simulink model "ParallelAssemblyEstimation2"  (R2024a)
settings: Solver=VariableStepAuto  StartTime=0.0  StopTime=10*10000  FixedStep=Ts  RelTol=1e-3  EnableMultiTasking=on
PreLoadFcn:
  | BatterySOHEstimationData;
values from neighbouring files (symbols this model uses):
  BalThreshold = 0.005    [ParallelAssemblyEstimationData.m]
  Ki = 10    [ParallelAssemblyEstimationData.m]
  Kp = 100    [ParallelAssemblyEstimationData.m]
  R = 0.05    [ParallelAssemblyEstimationData.m]
  R00 = 0.008    [ParallelAssemblyEstimationData.m]
  R0_mat = [.0117, .0085, .009; .011, .0085, .009; .0114, .0087, .0092; .0107, .0082, .0088; .0107, .0083, .0091; .0113, .0085, .0089; .0116, .0085, .0089]    [ParallelAssemblyEstimationData.m]
  SOC0 = initialSOC    (= 0.1)    [ParallelAssemblyEstimationData.m]
  Ts = 1    [ParallelAssemblyEstimationData.m]
libraries: nesl_utility x9, fl_lib x8, simulink x2, BatteryEstimators x2, BatteryCurrentManagement x1, BatteryBalancing x1, PouchCellAMP20M1HD x1, PouchCellAMP20M1HD_2 x1
CloseFcn:
  | try
  |     close(h1_BatterySOHEstimation)
  | catch
  | end
  | 
  | clear h1_BatterySOHEstimation
  | 
  | clear BatterySOHEstimationSimlog
  | clear BatterySOHEstimationLogsout
  | 
  | clear AH SOC_vec T_vec R0_mat R1_mat tau1_mat
  | clear V0_mat Q R P0 initialSOC SOC0 R00 Ts
  | clear cell_area h_conv thermal_mass
Description:
  | Battery State-of-Health Estimation
settings Model: Creator=The MathWorks, Inc.  LastModifiedBy=Carlos
settings SolverCC: AlgebraicLoopSolver=TrustRegion  AutoInsertRateTranBlk=on  MaxZcPerStep=1
settings DataIOCC: MaxDataPoints=370000  ReturnWorkspaceOutputs=off  SignalLoggingName=BatterySOHEstimationLogsout
settings OptimizationCC: ReuseModelBlockBuffer=off  LifeSpan=inf
settings DebuggingCC: UnconnectedInputMsg=warning  UnconnectedOutputMsg=warning  UnconnectedLineMsg=warning  SFUnexpectedBacktrackingDiag=warning  SFNoUnconditionalDefaultTransitionDiag=warning  SFExecutionAtInitializationDiag=none  ArithmeticOperatorsInVariantConditions=warning
settings ModelReferenceCC: EnableRefExpFcnMdlSchedulingChecks=on
settings SFSimCC: SimUseLocalCustomCode=off  CustomCodeUndefinedFunction=UseInterfaceOnly
settings RTWCC: RTWUseLocalCustomCode=off  GPUComputeCapability=3.5  DLArmComputeVersion=19.05
settings CodeAppCC: StateflowObjectComments=on
settings GRTTargetCC: TargetLangStandard=C89/C90 (ANSI)
settings ConfigComp: CovMetricSettings=dw  CovSaveCumulativeToWorkspaceVar=on  CovSaveSingleToWorkspaceVar=on  CovExternalEMLEnable=off
settings SimscapeCC: SimscapeLogType=all  SimscapeLogSimulationStatistics=on  SimscapeLogName=BatterySOHEstimationSimlog  SimscapeLogDataHistory=370000

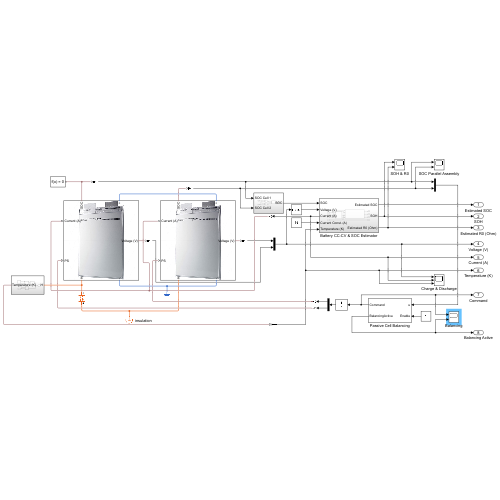
[thumbnail: Simulink's stored preview of the top-level diagram]
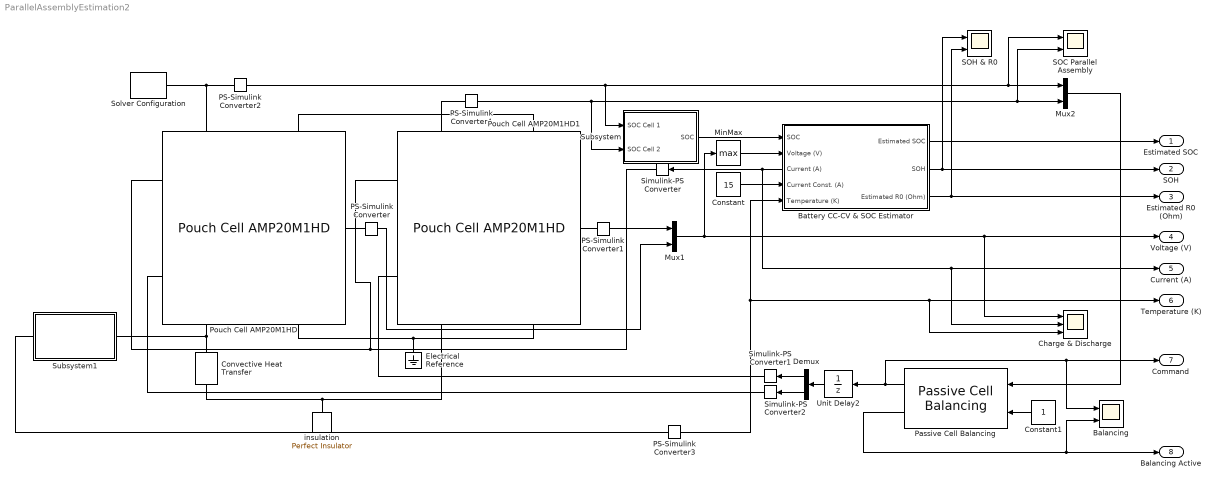
== system ParallelAssemblyEstimation2 ==
  Balancing : Scope  NumInputPorts=2
  Battery CC-CV & SOC Estimator : Subsystem
      settings: PortSchema="{\"entries\":[{\"content\":{\"sides\":[{\"content\":{\"connectorIds\":[\"In1\",\"In2\",\"Out4\",\"In3\",\"In4\"]},\"type\":\"ConnectorPlacement.EquallySpacedRectSide\",\"uuid\":\"2514b7b4-00c3-492f-9a2e-50aa1b82d6f8\"},{\"content\":{\"connectorIds\":[\"Out1\",\"Out2\",\"Out3\"],\"side\":\"RIGHT\"},\"type\":\"ConnectorPlacement.EquallySpacedRectSide\",\"uuid\":\"cd4e48b2-778c-43ee-9be2-ddbae3415521\"},{\"content\":{\"side\":\"TOP\"},\"type\":\"ConnectorPlacement.EquallySpacedRectSide\",\"uuid\":\"5acb0ed7-42f7-4cae-ae5e-6504fab96612\"}]},\"type\":\"ConnectorPlacement.EquallySpacedConnector\",\"uuid\":\"df921565-b99f-40a9-8d77-9b2ba5142a69\"}],\"packageUris\":[\"http://schema.mathworks.com/mf0/Connector/R2020b\"],\"version\":\"1.0\"}"
  Charge & Discharge : Scope  NumInputPorts=3
  Constant : Constant  Value=15
  Constant1 : Constant
  Convective Heat Transfer : fl_lib/Thermal/Thermal Elements/Convective Heat Transfer  thermal_type=foundation.enum.constant_variable.constant  area=cell_area m^2  heat_tr_coeff=h_conv W/(K*m^2)  min_heat_tr_coeff=1e-3 W/(K*m^2)  T_specify=off  T_priority=None  T=0 K  T_nominal_specify=off  T_nominal_value=1  T_nominal_unit=K  Q_specify=off  Q_priority=None  Q=0 W  Q_nominal_specify=off  Q_nominal_value=1  Q_nominal_unit=W
  Demux : Demux  Outputs=2
  Electrical Reference : fl_lib/Electrical/Electrical Elements/Electrical Reference
  MinMax : MinMax  Function=max
  Mux1 : Mux  Inputs=2
  Mux2 : Mux  Inputs=2
  PS-Simulink Converter{,1..4} (5 alike) : nesl_utility/PS-Simulink Converter  PhysicalDomain=network_engine_domain  SubClassName=ps_output  LeftPortType=input  RightPortType=output  PseudoPeriodic=off  Frequencies=[]  VectorFormat=inherit  Unit=inherit  AffineConversion=off
  Passive Cell Balancing : BatteryBalancing/Passive Cell Balancing  Threshold=BalThreshold  HysteresisBand=0  Td_on=1  Td_off=1  Ts=Ts  dataType=double
      settings: LibrarySourceBlock=batt_sl_lib/Cell Balancing/Passive Cell Balancing
  Pouch Cell AMP20M1HD : PouchCellAMP20M1HD/Pouch Cell AMP20M1HD  SystemSampleTime=-1  VariantActivationTime=update diagram  AllowFlexibleInterface=on  Latency=0  AutoFrameSizeCalculation=off
      settings: PortSchema="{\"entries\":[{\"content\":{\"sides\":[{\"content\":{\"connectorIds\":[\"LConn1\",\"LConn2\"]},\"type\":\"ConnectorPlacement.EquallySpacedRectSide\",\"uuid\":\"1ad4bd77-f3cd-4a33-b1f1-8549cde45efa\"},{\"content\":{\"connectorIds\":[\"RConn1\"],\"side\":\"RIGHT\"},\"type\":\"ConnectorPlacement.EquallySpacedRectSide\",\"uuid\":\"9571ac2f-f2ec-4c0a-999c-8ea72e2cf4ad\"},{\"content\":{\"connectorIds\":[\"LConn3\",\"LConn4\"],\"side\":\"TOP\"},\"type\":\"ConnectorPlacement.EquallySpacedRectSide\",\"uuid\":\"d345a9ac-e4a8-4cf5-b4f6-097232c3cb5c\"},{\"content\":{\"connectorIds\":[\"RConn2\",\"RConn3\"],\"side\":\"BOTTOM\"},\"type\":\"ConnectorPlacement.EquallySpacedRectSide\",\"uuid\":\"7baf50c1-841c-4e4e-b39d-add364b405c0\"}]},\"type\":\"ConnectorPlacement.EquallySpacedConnector\",\"uuid\":\"1a2d2ccb-b2c1-437b-8298-ee46cad3b357\"}],\"packageUris\":[\"http://schema.mathworks.com/mf0/Connector/R2020b\"],\"version\":\"1.0\"}"
  Pouch Cell AMP20M1HD1 : PouchCellAMP20M1HD_2/Pouch Cell AMP20M1HD  SystemSampleTime=-1  VariantActivationTime=update diagram  AllowFlexibleInterface=on  Latency=0  AutoFrameSizeCalculation=off
      settings: PortSchema="{\"entries\":[{\"content\":{\"sides\":[{\"content\":{\"connectorIds\":[\"LConn1\",\"LConn2\"]},\"type\":\"ConnectorPlacement.EquallySpacedRectSide\",\"uuid\":\"1ad4bd77-f3cd-4a33-b1f1-8549cde45efa\"},{\"content\":{\"connectorIds\":[\"RConn1\"],\"side\":\"RIGHT\"},\"type\":\"ConnectorPlacement.EquallySpacedRectSide\",\"uuid\":\"9571ac2f-f2ec-4c0a-999c-8ea72e2cf4ad\"},{\"content\":{\"connectorIds\":[\"LConn3\",\"LConn4\"],\"side\":\"TOP\"},\"type\":\"ConnectorPlacement.EquallySpacedRectSide\",\"uuid\":\"d345a9ac-e4a8-4cf5-b4f6-097232c3cb5c\"},{\"content\":{\"connectorIds\":[\"RConn2\",\"RConn3\"],\"side\":\"BOTTOM\"},\"type\":\"ConnectorPlacement.EquallySpacedRectSide\",\"uuid\":\"7baf50c1-841c-4e4e-b39d-add364b405c0\"}]},\"type\":\"ConnectorPlacement.EquallySpacedConnector\",\"uuid\":\"1a2d2ccb-b2c1-437b-8298-ee46cad3b357\"}],\"packageUris\":[\"http://schema.mathworks.com/mf0/Connector/R2020b\"],\"version\":\"1.0\"}"
  SOC Parallel Assembly : Scope  NumInputPorts=2
  SOH & R0 : Scope  NumInputPorts=2
  Simulink-PS Converter : nesl_utility/Simulink-PS Converter  PhysicalDomain=network_engine_domain  SubClassName=ps_input  LeftPortType=input  RightPortType=output  PseudoPeriodic=off  Frequencies=[]  NoiseDistribution=none  NoiseParameters=[]  Unit=1  AffineConversion=off  FilteringAndDerivatives=provide  SimscapeFilterOrder=1  InputFilterTimeConstant=0.001  UdotUserProvided=0
  Simulink-PS Converter1 : nesl_utility/Simulink-PS Converter  PhysicalDomain=network_engine_domain  SubClassName=ps_input  LeftPortType=input  RightPortType=output  PseudoPeriodic=off  Frequencies=[]  NoiseDistribution=none  NoiseParameters=[]  Unit=1  AffineConversion=off  FilteringAndDerivatives=provide  SimscapeFilterOrder=1  InputFilterTimeConstant=0.001  UdotUserProvided=0
  Simulink-PS Converter2 : nesl_utility/Simulink-PS Converter  PhysicalDomain=network_engine_domain  SubClassName=ps_input  LeftPortType=input  RightPortType=output  PseudoPeriodic=off  Frequencies=[]  NoiseDistribution=none  NoiseParameters=[]  Unit=1  AffineConversion=off  FilteringAndDerivatives=provide  SimscapeFilterOrder=1  InputFilterTimeConstant=0.001  UdotUserProvided=0
  Solver Configuration : nesl_utility/Solver Configuration  PhysicalDomain=network_engine_domain  SubClassName=solver  LeftPortType=input  RightPortType=generic  Tones=[]  Harmonics=[]  SimulateNoise=off  Profile=off  UseLocalSampling=off  EnableSwitchedLinearOptims=on  FrequencyDomain=off  UseCCode=off  RelTol=0.001  AbsTol=0.001  MinStep=1e-09  ToWorkspace=off  RevertToSquareIcSolve=off  NumHomotopyIterations=100  PhasorMode=off  PhasorModeNumHarmonics=1  ConsistencySolver=NEWTON_XTOL_AFTER_FTOL  IndexReductionMethod=DerivativeReplacement  DoDC=off  ResidualTolerance=1e-09  ConsistencyTolSource=GLOBAL  ConsistencyAbsTol=0.001  ConsistencyRelTol=0.001  ConsistencyTolFactor=0.001  UseLocalSolver=on  LocalSolverChoice=NE_BACKWARD_EULER_ADVANCER  ResolveIndetEquations=on  FunctionEvalNumThread=1  LocalSolverSampleTime=Ts  DoFixedCost=on  MaxNonlinIter=3  MaxModeIter=2  ComputeImpulses=off  ImpulseIterations=2  LinearAlgebra=auto  LinearAlgebraNumThread=0  EquationFormulation=NE_TIME_EF  DelaysMemoryBudget=1024  AutomaticFiltering=on  FilteringTimeConstant=0.001  PartitionStorageMethod=AS_NEEDED  PartitionMemoryBudget=1024  PartitionMethod=ROBUST  MultibodyUseLocalSolver=off  MultibodyLocalSolverChoice=ODE1  MultibodyLocalSolverSampleTime=0.001
  Subsystem : Subsystem
  Subsystem1 : Subsystem
  Unit Delay2 : UnitDelay  SampleTime=-1  HasFrameUpgradeWarning=on
  insulation : fl_lib/Thermal/Thermal Elements/Perfect Insulator  T_specify=off  T_priority=None  T=0 K  T_nominal_specify=off  T_nominal_value=1  T_nominal_unit=K
  Estimated SOC : Outport
  SOH : Outport  Port=2
  Estimated R0 (Ohm) : Outport  Port=3
  Voltage (V) : Outport  Port=4
  Current (A) : Outport  Port=5
  Temperature (K) : Outport  Port=6
  Command : Outport  Port=7
  Balancing Active : Outport  Port=8
  wires:
  Battery CC-CV & SOC Estimator/2(SOH) -> SOH/1, SOH & R0/1
  Battery CC-CV & SOC Estimator/3(Estimated R0 (Ohm)) -> Estimated R0 (Ohm)/1, SOH & R0/2
  Battery CC-CV & SOC Estimator/1(Estimated SOC) -> Estimated SOC/1
  Constant/1 -> Battery CC-CV & SOC Estimator/3(Current Const. (A))
  Battery CC-CV & SOC Estimator/4(Current (A)) -> Simulink-PS Converter/1, Charge & Discharge/2, Current (A)/1
  PS-Simulink Converter/1 -> Mux1/2
  Mux1/1 -> MinMax/1, Voltage (V)/1, Charge & Discharge/1
  PS-Simulink Converter4/1 -> Mux2/2, SOC Parallel Assembly/2, Subsystem/2(SOC Cell 2)
  PS-Simulink Converter2/1 -> SOC Parallel Assembly/1, Mux2/1, Subsystem/1(SOC Cell 1)
  Unit Delay2/1 -> Demux/1
  Passive Cell Balancing/1 -> Unit Delay2/1, Command/1, Balancing/1
  Passive Cell Balancing/2 -> Balancing Active/1, Balancing/2
  Demux/1 -> Simulink-PS Converter1/1
  Demux/2 -> Simulink-PS Converter2/1
  Constant1/1 -> Passive Cell Balancing/2
  MinMax/1 -> Battery CC-CV & SOC Estimator/2(Voltage (V))
  PS-Simulink Converter3/1 -> Temperature (K)/1, Charge & Discharge/3, Battery CC-CV & SOC Estimator/4(Temperature (K))
  PS-Simulink Converter1/1 -> Mux1/1
  Mux2/1 -> Passive Cell Balancing/1
  Subsystem/1(SOC) -> Battery CC-CV & SOC Estimator/1(SOC)
  connections:
  Pouch Cell AMP20M1HD/LConn4 -- Pouch Cell AMP20M1HD1/LConn4
  Electrical Reference/LConn1 -- Pouch Cell AMP20M1HD1/RConn3 -- Pouch Cell AMP20M1HD/RConn3
  Pouch Cell AMP20M1HD/RConn1 -- PS-Simulink Converter/LConn1
  PS-Simulink Converter1/LConn1 -- Pouch Cell AMP20M1HD1/RConn1
  PS-Simulink Converter2/LConn1 -- Solver Configuration/RConn1 -- Pouch Cell AMP20M1HD/LConn3
  PS-Simulink Converter4/LConn1 -- Pouch Cell AMP20M1HD1/LConn3
  Simulink-PS Converter/RConn1 -- Pouch Cell AMP20M1HD1/LConn1 -- Pouch Cell AMP20M1HD/LConn1
  Pouch Cell AMP20M1HD/RConn2 -- Convective Heat Transfer/LConn1 -- Subsystem1/RConn1
  Pouch Cell AMP20M1HD1/LConn2 -- Simulink-PS Converter1/RConn1
  Pouch Cell AMP20M1HD/LConn2 -- Simulink-PS Converter2/RConn1
  PS-Simulink Converter3/LConn1 -- Subsystem1/LConn1
  insulation/LConn1 -- Pouch Cell AMP20M1HD1/RConn2 -- Convective Heat Transfer/RConn1

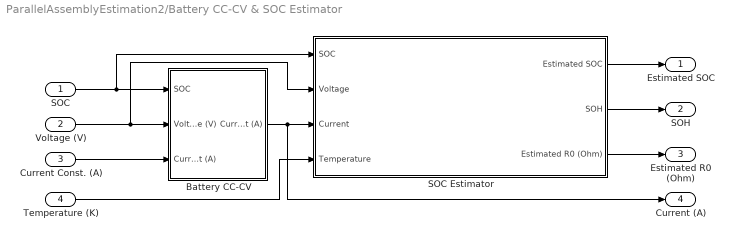
== system ParallelAssemblyEstimation2/Battery CC-CV & SOC Estimator ==
  SOC : Inport
  Voltage (V) : Inport  Port=2
  Current Const. (A) : Inport  Port=3
  Temperature (K) : Inport  Port=4
  Battery CC-CV : Subsystem
  SOC Estimator : Subsystem
  Estimated SOC : Outport
  SOH : Outport  Port=2
  Estimated R0 (Ohm) : Outport  Port=3
  Current (A) : Outport  Port=4
  wires:
  Temperature (K)/1 -> SOC Estimator/4(Temperature)
  Battery CC-CV/1(Current Out (A)) -> SOC Estimator/3(Current), Current (A)/1
  SOC Estimator/2(SOH) -> SOH/1
  SOC Estimator/3(Estimated R0 (Ohm)) -> Estimated R0 (Ohm)/1
  SOC Estimator/1(Estimated SOC) -> Estimated SOC/1
  Current Const. (A)/1 -> Battery CC-CV/3(Current (A))
  Voltage (V)/1 -> SOC Estimator/2(Voltage), Battery CC-CV/2(Voltage (V))
  SOC/1 -> SOC Estimator/1(SOC), Battery CC-CV/1(SOC)

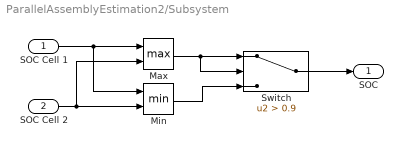
== system ParallelAssemblyEstimation2/Subsystem ==
  SOC Cell 1 : Inport
  SOC Cell 2 : Inport  Port=2
  Max : MinMax  Function=max  Inputs=2
  Min : MinMax  Inputs=2
  Switch : Switch  Criteria=u2 > Threshold  Threshold=0.9  SaturateOnIntegerOverflow=off  InputSameDT=off
  SOC : Outport
  wires:
  SOC Cell 1/1 -> Max/1, Min/1
  Max/1 -> Switch/1, Switch/2
  Min/1 -> Switch/3
  SOC Cell 2/1 -> Max/2, Min/2
  Switch/1 -> SOC/1

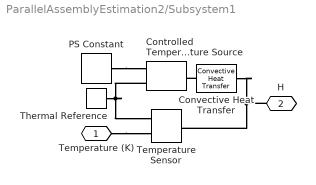
== system ParallelAssemblyEstimation2/Subsystem1 ==
  Controlled Temperature Source : fl_lib/Thermal/Thermal Sources/Controlled Temperature Source
  Convective Heat Transfer : fl_lib/Thermal/Thermal Elements/Convective Heat Transfer  thermal_type=foundation.enum.constant_variable.constant  area=cell_area m^2  heat_tr_coeff=h_conv W/(K*m^2)  min_heat_tr_coeff=1e-3 W/(K*m^2)  T_specify=off  T_priority=None  T=0 K  T_nominal_specify=off  T_nominal_value=1  T_nominal_unit=K  Q_specify=off  Q_priority=None  Q=0 W  Q_nominal_specify=off  Q_nominal_value=1  Q_nominal_unit=W
  PS Constant : fl_lib/Physical Signals/Sources/PS Constant  constant=cell_temperature K
  Temperature Sensor : fl_lib/Thermal/Thermal Sensors/Temperature Sensor  temperature_measure=foundation.enum.MeasurementReference.difference
  Thermal Reference : fl_lib/Thermal/Thermal Elements/Thermal Reference
  Temperature (K) : PMIOPort  Side=Left
  H : PMIOPort  Port=2  Side=Right
  connections:
  H/RConn1 -- Convective Heat Transfer/RConn1 -- Temperature Sensor/LConn1
  Thermal Reference/LConn1 -- Controlled Temperature Source/RConn2 -- Temperature Sensor/RConn1
  PS Constant/RConn1 -- Controlled Temperature Source/RConn1
  Temperature (K)/RConn1 -- Temperature Sensor/RConn2
  Convective Heat Transfer/LConn1 -- Controlled Temperature Source/LConn1

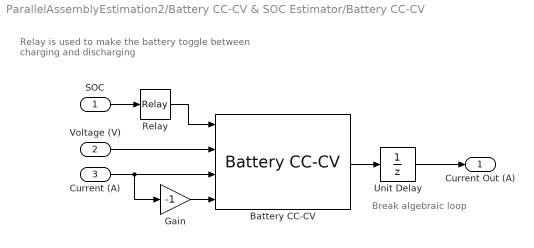
== system ParallelAssemblyEstimation2/Battery CC-CV & SOC Estimator/Battery CC-CV ==
  note: Break algebraic loop
  note: Relay is used to make the battery toggle between charging and discharging
  SOC : Inport
  Voltage (V) : Inport  Port=2
  Current (A) : Inport  Port=3
  Battery CC-CV : BatteryCurrentManagement/Battery CC-CV  MaxCellVoltage=vMax  Kp=Kp  Ki=Ki  Kaw=Kaw  Kt=1  Ts=Ts
      settings: LibrarySourceBlock=batt_sl_lib/Current Management/Battery CC-CV
  Gain : Gain  Gain=-1
  Relay : Relay  OnSwitchValue=0.9186  OffSwitchValue=0.3  OnOutputValue=0  OffOutputValue=1
  Unit Delay : UnitDelay  SampleTime=-1  HasFrameUpgradeWarning=on
  Current Out (A) : Outport
  wires:
  Voltage (V)/1 -> Battery CC-CV/2
  Battery CC-CV/1 -> Unit Delay/1
  Relay/1 -> Battery CC-CV/1
  SOC/1 -> Relay/1
  Gain/1 -> Battery CC-CV/4
  Current (A)/1 -> Gain/1, Battery CC-CV/3
  Unit Delay/1 -> Current Out (A)/1

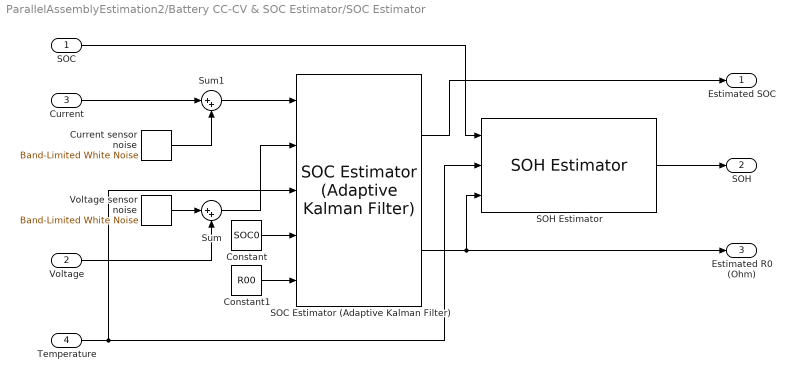
== system ParallelAssemblyEstimation2/Battery CC-CV & SOC Estimator/SOC Estimator ==
  SOC : Inport
  Voltage : Inport  Port=2
  Current : Inport  Port=3
  Temperature : Inport  Port=4
  Constant : Constant  Value=SOC0
  Constant1 : Constant  Value=R00
  Current sensor noise : simulink/Sources/Band-Limited White Noise  Cov=1e-3  Ts=1  seed=1
  SOC Estimator (Adaptive Kalman Filter) : BatteryEstimators/SOC Estimator (Adaptive Kalman Filter)  CurrentInputPartition=off  filterType=Unscented Kalman filter  alpha=1  beta=2  kappa=0  Q=Q  Q_2RC=|  R=R  P0=P0  P0_2RC="[1e-5 0 0 0; 0 1 0 0;0 0  1 0; 0 0 0 1e-5]"  Ts=Ts  chargeDynamics=One time-constant dynamics  SOC_vec=SOC_vec  T_vec=T_vec  R1_mat=R1_mat  tau1_mat=tau1_mat  R2_mat=[.0109, .0029, .0013; .0069, .0024, .0012; .0047, .0026, .0013; .0034, .0016, .001; .0033, .0023, .0014; .0033, .0018, .0011; .0028, .0017, .0011]  tau2_mat=[20, 36, 39; 31, 45, 39; 109, 105, 61; 36, 29, 26; 59, 77, 67; 40, 33, 29; 25, 39, 33]  V0_mat=V0_mat  AH=AH
      | [1e-6 0 0 0;
      | 0 1e-6 0 0;0 0 1e-6 0;0 0 0 1e-6]
  SOH Estimator : BatteryEstimators/SOH Estimator  SOC_vec=SOC_vec  T_vec=T_vec  R0_new_mat=R0_mat  R0_EOL_mat=R0_mat*3
  Sum : Sum  Inputs=|++
  Sum1 : Sum  Inputs=|++
  Voltage sensor noise : simulink/Sources/Band-Limited White Noise  Cov=1e-3  Ts=1  seed=23341
  Estimated SOC : Outport
  SOH : Outport  Port=2
  Estimated R0 (Ohm) : Outport  Port=3
  wires:
  SOC Estimator (Adaptive Kalman Filter)/1 -> Estimated SOC/1
  Sum/1 -> SOC Estimator (Adaptive Kalman Filter)/2
  Voltage sensor noise/1 -> Sum/1
  Constant1/1 -> SOC Estimator (Adaptive Kalman Filter)/5
  SOC Estimator (Adaptive Kalman Filter)/2 -> Estimated R0 (Ohm)/1, SOH Estimator/3
  Constant/1 -> SOC Estimator (Adaptive Kalman Filter)/4
  Sum1/1 -> SOC Estimator (Adaptive Kalman Filter)/1
  Voltage/1 -> Sum/2
  Current sensor noise/1 -> Sum1/2
  Temperature/1 -> SOH Estimator/2, SOC Estimator (Adaptive Kalman Filter)/3
  SOH Estimator/1 -> SOH/1
  Current/1 -> Sum1/1
  SOC/1 -> SOH Estimator/1
